simulink model "sistema_completo_discretizado"  (R2023b)
settings: Solver=VariableStepAuto  StartTime=0.0  StopTime=10.0  RelTol=1e-3
values from neighbouring files (symbols this model uses):
  alpha_Cu = 3.9e-3    (= 0.0039)    [controlador_foc_simulink.m]    (also in parametros_planta.m; params_subsistema_termico.m; sistema_completo_en_codigo.m)
  ba_num = Jeq_ctrl*n_pid*wn_pid    (= 0.0395694444444)    [controlador_foc_simulink.m]    (also in sistema_completo_en_codigo.m)
  beq_nom = bm + bl_nom/r^2    (= 2.19444444444e-05)    [parametros_planta.m]    (also in params_subsistema_mecanico.m; sistema_completo_en_codigo.m)
  Cts = 0.818    [parametros_planta.m]    (also in params_subsistema_termico.m)
  g = 9.80665    [controlador_foc_simulink.m]    (also in parametros_planta.m; params_subsistema_mecanico.m; sistema_completo_en_codigo.m)
  Jeq_nom = Jm + Jl_nom/r^2    (= 1.97847222222e-05)    [params_subsistema_mecanico.m]    (also in sistema_completo_en_codigo.m)
  kg_eq_nom = g*kl_nom/r    (= 0.0204305208333)    [params_subsistema_mecanico.m]    (also in sistema_completo_en_codigo.m)
  kl_nom = m*Lcm + ml_nom*Ll    (= 0.25)    [controlador_foc_simulink.m]    (also in params_subsistema_mecanico.m; sistema_completo_en_codigo.m)
  Ksa_num = Jeq_ctrl*n_pid*wn_pid^2    (= 31.6555555556)    [controlador_foc_simulink.m]    (also in sistema_completo_en_codigo.m)
  Ksia_num = Jeq_ctrl*wn_pid^3    (= 10129.7777778)    [controlador_foc_simulink.m]    (also in sistema_completo_en_codigo.m)
  L_d = 6.6e-3    (= 0.0066)    [controlador_foc_simulink.m]    (also in params_subsistema_electromagnetico.m; sistema_completo_en_codigo.m)
  L_l = 0.8e-3    (= 0.0008)    [controlador_foc_simulink.m]    (also in params_subsistema_electromagnetico.m; sistema_completo_en_codigo.m)
  L_q = 5.8e-3    (= 0.0058)    [controlador_foc_simulink.m]    (also in params_subsistema_electromagnetico.m; sistema_completo_en_codigo.m)
  lambda_m = 0.016    [controlador_foc_simulink.m]    (also in parametros_planta.m; params_subsistema_electromagnetico.m; sistema_completo_en_codigo.m)
  Pp = 3    [controlador_foc_simulink.m]    (also in parametros_planta.m; params_subsistema_electromagnetico.m; sistema_completo_en_codigo.m)
  r = 120.0    (= 120)    [controlador_foc_simulink.m]    (also in parametros_planta.m; params_subsistema_mecanico.m; sistema_completo_en_codigo.m)
  Rs_REF = 1.02    [controlador_foc_simulink.m]    (also in parametros_planta.m; params_subsistema_termico.m; sistema_completo_en_codigo.m)
  Rts_amb = 146.7    [parametros_planta.m]    (also in params_subsistema_termico.m)
  Tamb = Tamb_max    (= 40)    [parametros_planta.m]    (also in params_subsistema_termico.m; sistema_completo_en_codigo.m)
  Ts = interp_ts(Ts_ts,t)    [calcular_metricas_operacion.m]
  Ts_REF = 20.0    (= 20)    [controlador_foc_simulink.m]    (also in parametros_planta.m; params_subsistema_termico.m; sistema_completo_en_codigo.m)
undefined symbols (not defined in the file or in its folder): A_iabc, A_pos, A_T, A_v, B_iabc, B_pos, B_T, B_v, C_iabc, C_pos, C_T, C_v, D_iabc, D_pos, D_T, D_v, DiscIntNeverNeededParam, K_ei_ext_agresivo, K_eth_ext_agresivo, K_ew_ext_agresivo
settings Model: Creator=Pc  LastModifiedBy=Pc

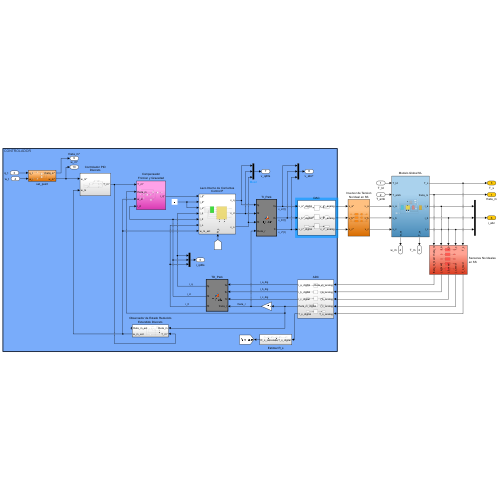
[thumbnail: Simulink's stored preview of the top-level diagram]
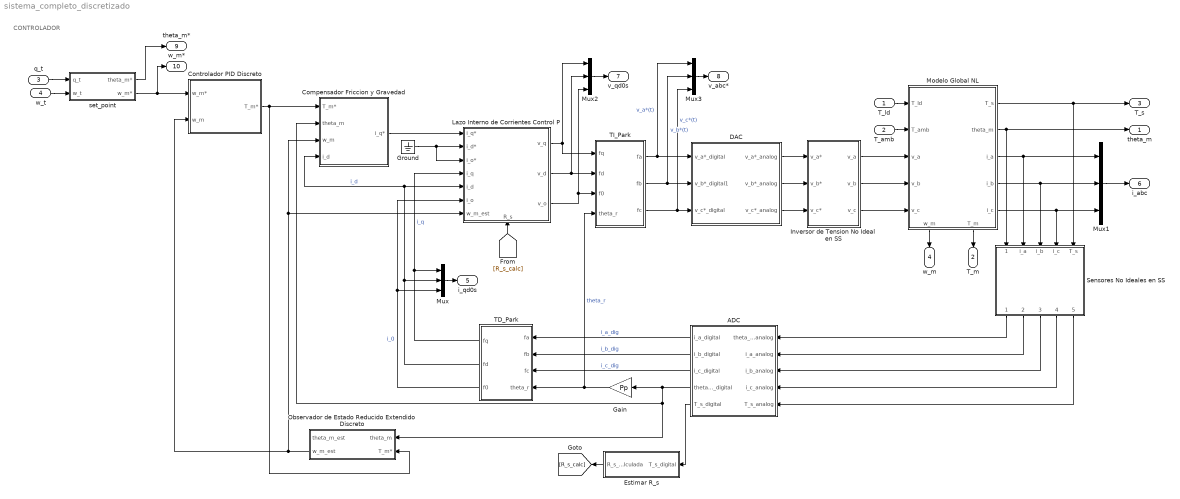
== system sistema_completo_discretizado ==
  note: CONTROLADOR
  T_ld : Inport
  T_amb : Inport  Port=2
  q_t : Inport  Port=3
  w_t : Inport  Port=4
  " ADC" : Subsystem
  Compensador Friccion y Gravedad : Subsystem
  Controlador PID Discreto : Subsystem
  DAC : Subsystem
  Estimar R_s : Subsystem
  Gain : Gain  Gain=Pp
  Ground : Ground
  Inversor de Tension No Ideal en SS : Subsystem
  Lazo Interno de Corrientes Control P : Subsystem
      settings: PortSchema="{\"entries\":[{\"content\":{\"sides\":[{\"content\":{\"connectorIds\":[\"In1\",\"In2\",\"In3\",\"In4\",\"In5\",\"In6\",\"In7\"]},\"type\":\"ConnectorPlacement.EquallySpacedRectSide\",\"uuid\":\"003130de-7086-42b2-88ab-1550be464119\"},{\"content\":{\"connectorIds\":[\"Out1\",\"Out2\",\"Out3\"],\"side\":\"RIGHT\"},\"type\":\"ConnectorPlacement.EquallySpacedRectSide\",\"uuid\":\"1ef26d10-ae91-4351-8dbc-50b579db1e66\"},{\"content\":{\"side\":\"TOP\"},\"type\":\"ConnectorPlacement.EquallySpacedRectSide\",\"uuid\":\"f8d5b360-b304-4c62-a3c0-e85b3671d199\"},{\"content\":{\"connectorIds\":[\"In8\"],\"side\":\"BOTTOM\"},\"type\":\"ConnectorPlacement.EquallySpacedRectSide\",\"uuid\":\"ca7bddea-434a-49b1-aeae-36f1f1b68346\"}]},\"type\":\"ConnectorPlacement.EquallySpacedConnector\",\"uuid\":\"97d0594b-d096-4b47-8675-ea576c5ffe32\"}],\"packageUris\":[\"http://schema.mathworks.com/mf0/Connector/R2020b\"],\"version\":\"1.0\"}"
  Modelo Global NL : Subsystem
      settings: PortSchema="{\"entries\":[{\"content\":{\"sides\":[{\"content\":{\"connectorIds\":[\"In1\",\"In2\",\"In3\",\"In4\",\"In5\"]},\"type\":\"ConnectorPlacement.EquallySpacedRectSide\",\"uuid\":\"386252be-5f39-4928-a151-52e681895a84\"},{\"content\":{\"connectorIds\":[\"Out1\",\"Out2\",\"Out3\",\"Out4\",\"Out5\"],\"side\":\"RIGHT\"},\"type\":\"ConnectorPlacement.EquallySpacedRectSide\",\"uuid\":\"aee83b90-e95b-4477-b157-a5534e7c5e6c\"},{\"content\":{\"side\":\"TOP\"},\"type\":\"ConnectorPlacement.EquallySpacedRectSide\",\"uuid\":\"e739b3f7-cae1-4498-b396-d13f7405e232\"},{\"content\":{\"connectorIds\":[\"Out6\",\"Out7\"],\"side\":\"BOTTOM\"},\"type\":\"ConnectorPlacement.EquallySpacedRectSide\",\"uuid\":\"86304fed-22cd-46a2-87e5-e7bae1c5cedf\"}]},\"type\":\"ConnectorPlacement.EquallySpacedConnector\",\"uuid\":\"c0eb110b-b212-4702-a1d5-9ec3ac2ff196\"}],\"packageUris\":[\"http://schema.mathworks.com/mf0/Connector/R2020b\"],\"version\":\"1.0\"}"
  Mux{,1..3} (4 alike) : Mux  Inputs=3
  Observador de Estado Reducido Extendido Discreto : Subsystem
  Sensores No Ideales en SS : Subsystem
  TD_Park : MATLAB Function  TreatAsAtomicUnit=on
  TI_Park : MATLAB Function  TreatAsAtomicUnit=on
  set_point : Subsystem
  theta_m : Outport
  T_m : Outport  Port=2
  T_s : Outport  Port=3
  w_m : Outport  Port=4
  i_qd0s : Outport  Port=5
  i_abc : Outport  Port=6
  v_qd0s : Outport  Port=7
  v_abc* : Outport  Port=8
  theta_m* : Outport  Port=9
  w_m* : Outport  Port=10
  wires:
  Inversor de Tension No Ideal en SS/3(v_c) -> Modelo Global NL/5(v_c)
  w_t/1 -> set_point/2(w_t)
  Modelo Global NL/6(w_m) -> w_m/1
  q_t/1 -> set_point/1(q_t)
  Mux1/1 -> i_abc/1
  Ground/1 -> Lazo Interno de Corrientes Control P/3(i_o*), Lazo Interno de Corrientes Control P/2(i_d*)
  T_ld/1 -> Modelo Global NL/1(T_ld)
  TI_Park/2(fb) -> DAC/2(v_b*_digital1), Mux3/2  "v_b*(t)"
  TD_Park/3(f0) -> Mux/3, Lazo Interno de Corrientes Control P/6(i_o)  "i_0"
  Modelo Global NL/3(i_a) -> Mux1/1, Sensores No Ideales en SS/2(i_a)
  TI_Park/3(fc) -> DAC/3(v_c*_digital), Mux3/3  "v_c*(t)"
  T_amb/1 -> Modelo Global NL/2(T_amb)
  Modelo Global NL/5(i_c) -> Mux1/3, Sensores No Ideales en SS/4(i_c)
  Mux3/1 -> v_abc*/1
  TD_Park/1(fq) -> Mux/1, Lazo Interno de Corrientes Control P/4(i_q)  "i_q"
  Sensores No Ideales en SS/1(theta_m_med) -> " ADC"/1(theta_m_analog)
  Gain/1 -> TD_Park/4(theta_r), TI_Park/4(theta_r)  "theta_r"
  Modelo Global NL/4(i_b) -> Mux1/2, Sensores No Ideales en SS/3(i_b)
  set_point/1(theta_m*) -> theta_m*/1
  Inversor de Tension No Ideal en SS/1(v_a) -> Modelo Global NL/3(v_a)
  Modelo Global NL/7(T_m) -> T_m/1
  Mux2/1 -> v_qd0s/1
  TI_Park/1(fa) -> DAC/1(v_a*_digital), Mux3/1  "v_a*(t)"
  TD_Park/2(fd) -> Compensador Friccion y Gravedad/4(i_d), Lazo Interno de Corrientes Control P/5(i_d), Mux/2  "i_d"
  Mux/1 -> i_qd0s/1
  Inversor de Tension No Ideal en SS/2(v_b) -> Modelo Global NL/4(v_b)
  Modelo Global NL/1(T_s) -> Sensores No Ideales en SS/5(T_s), T_s/1
  Modelo Global NL/2(theta_m) -> theta_m/1, Sensores No Ideales en SS/1(theta_m)
  Sensores No Ideales en SS/2(i_a_med) -> " ADC"/2(i_a_analog)
  Sensores No Ideales en SS/3(i_b_med) -> " ADC"/3(i_b_analog)
  Sensores No Ideales en SS/4(i_c_med) -> " ADC"/4(i_c_analog)
  DAC/3(v_c*_analog) -> Inversor de Tension No Ideal en SS/3(v_c*)
  DAC/2(v_b*_analog) -> Inversor de Tension No Ideal en SS/2(v_b*)
  DAC/1(v_a*_analog) -> Inversor de Tension No Ideal en SS/1(v_a*)
  " ADC"/1(i_a_digital) -> TD_Park/1(fa)  "i_a_dig"
  " ADC"/2(i_b_digital) -> TD_Park/2(fb)  "i_b_dig"
  " ADC"/3(i_c_digital) -> TD_Park/3(fc)  "i_c_dig"
  Sensores No Ideales en SS/5(T_s_med) -> " ADC"/5(T_s_analog)
  Lazo Interno de Corrientes Control P/1(v_q) -> TI_Park/1(fq), Mux2/1
  Lazo Interno de Corrientes Control P/2(v_d) -> TI_Park/2(fd), Mux2/2
  Lazo Interno de Corrientes Control P/3(v_o) -> TI_Park/3(f0), Mux2/3
  Compensador Friccion y Gravedad/1(i_q*) -> Lazo Interno de Corrientes Control P/1(i_q*)
  " ADC"/5(T_s_digital) -> Estimar R_s/1(T_s_digital)
  [R_s_calc] -> Lazo Interno de Corrientes Control P/8(R_s)
  Estimar R_s/1(R_s_calculada) -> [R_s_calc]
  Controlador PID Discreto/1(T_m*) -> Observador de Estado Reducido Extendido Discreto/2(T_m*), Compensador Friccion y Gravedad/1(T_m*)
  set_point/2(w_m*) -> Controlador PID Discreto/1(w_m*), w_m*/1
  Observador de Estado Reducido Extendido Discreto/2(w_m_est) -> Controlador PID Discreto/2(w_m), Lazo Interno de Corrientes Control P/7(w_m_est), Compensador Friccion y Gravedad/3(w_m)
  " ADC"/4(theta_m_digital) -> Gain/1, Observador de Estado Reducido Extendido Discreto/1(theta_m), Compensador Friccion y Gravedad/2(theta_m)

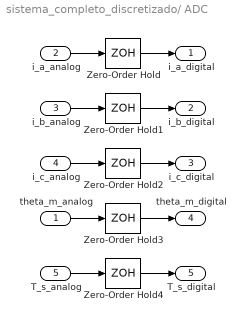
== system sistema_completo_discretizado/ ADC ==
  theta_m_analog : Inport
  i_a_analog : Inport  Port=2
  i_b_analog : Inport  Port=3
  i_c_analog : Inport  Port=4
  T_s_analog : Inport  Port=5
  Zero-Order Hold{,1..4} (5 alike) : ZeroOrderHold  SampleTime=Ts
  i_a_digital : Outport
  i_b_digital : Outport  Port=2
  i_c_digital : Outport  Port=3
  theta_m_digital : Outport  Port=4
  T_s_digital : Outport  Port=5
  wires:
  theta_m_analog/1 -> Zero-Order Hold3/1
  i_a_analog/1 -> Zero-Order Hold/1
  Zero-Order Hold/1 -> i_a_digital/1
  i_c_analog/1 -> Zero-Order Hold2/1
  i_b_analog/1 -> Zero-Order Hold1/1
  T_s_analog/1 -> Zero-Order Hold4/1
  Zero-Order Hold1/1 -> i_b_digital/1
  Zero-Order Hold2/1 -> i_c_digital/1
  Zero-Order Hold3/1 -> theta_m_digital/1
  Zero-Order Hold4/1 -> T_s_digital/1

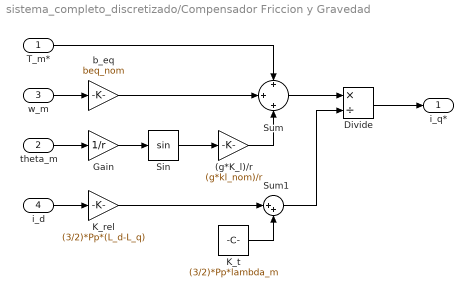
== system sistema_completo_discretizado/Compensador Friccion y Gravedad ==
  T_m* : Inport
  theta_m : Inport  Port=2
  w_m : Inport  Port=3
  i_d : Inport  Port=4
  (g*K_l)/r : Gain  Gain=(g*kl_nom)/r
  Divide : Product  Inputs=*/
  Gain : Gain  Gain=1/r
  K_rel : Gain  Gain=(3/2)*Pp*(L_d-L_q)
  K_t : Constant  Value=(3/2)*Pp*lambda_m
  Sin : Trigonometry
  Sum : Sum  Inputs=+|+|+
  Sum1 : Sum  Inputs=|++
  b_eq : Gain  Gain=beq_nom
  i_q* : Outport
  wires:
  i_d/1 -> K_rel/1
  T_m*/1 -> Sum/1
  Sin/1 -> (g*K_l)/r/1
  K_t/1 -> Sum1/2
  (g*K_l)/r/1 -> Sum/3
  Sum1/1 -> Divide/2
  Gain/1 -> Sin/1
  b_eq/1 -> Sum/2
  K_rel/1 -> Sum1/1
  w_m/1 -> b_eq/1
  Sum/1 -> Divide/1
  Divide/1 -> i_q*/1
  theta_m/1 -> Gain/1

== system sistema_completo_discretizado/Controlador PID Discreto ==
  w_m* : Inport
  w_m : Inport  Port=2
  Discrete-Time Integrator : DiscreteIntegrator  IntegratorMethod=Integration: Trapezoidal  SampleTime=-1  ICPrevOutput=DiscIntNeverNeededParam  ICPrevScaledInput=DiscIntNeverNeededParam
  Discrete-Time Integrator1 : DiscreteIntegrator  IntegratorMethod=Integration: Trapezoidal  SampleTime=-1  ICPrevOutput=DiscIntNeverNeededParam  ICPrevScaledInput=DiscIntNeverNeededParam
  Ksa : Gain  Gain=Ksa_num
  Ksia : Gain  Gain=Ksia_num
  Sum : Sum  Inputs=++|
  Sum1 : Sum  Inputs=+|+|+
  ba : Gain  Gain=ba_num
  T_m* : Outport
  wires:
  Sum1/1 -> T_m*/1
  ba/1 -> Sum1/3  "D"
  Sum/1 -> ba/1, Discrete-Time Integrator/1  "err_w_m"
  Discrete-Time Integrator1/1 -> Ksia/1
  w_m*/1 -> Sum/1
  Discrete-Time Integrator/1 -> Ksa/1, Discrete-Time Integrator1/1
  w_m/1 -> Sum/2
  Ksia/1 -> Sum1/1  "I"
  Ksa/1 -> Sum1/2  "P"

== system sistema_completo_discretizado/DAC ==
  v_a*_digital : Inport
  v_b*_digital1 : Inport  Port=2
  v_c*_digital : Inport  Port=3
  First Order Hold1 : FirstOrderHold  ErrorTolerance=inf  AllowContinuousInput=on
  First Order Hold2 : FirstOrderHold  ErrorTolerance=inf  AllowContinuousInput=on
  First Order Hold4 : FirstOrderHold  ErrorTolerance=inf  AllowContinuousInput=on
  v_a*_analog : Outport
  v_b*_analog : Outport  Port=2
  v_c*_analog : Outport  Port=3
  wires:
  v_c*_digital/1 -> First Order Hold2/1
  v_b*_digital1/1 -> First Order Hold1/1
  v_a*_digital/1 -> First Order Hold4/1
  First Order Hold4/1 -> v_a*_analog/1
  First Order Hold1/1 -> v_b*_analog/1
  First Order Hold2/1 -> v_c*_analog/1

== system sistema_completo_discretizado/Estimar R_s ==
  T_s_digital : Inport
  Constant3 : Constant
  Rs_ref : Gain  Gain=Rs_REF
  Sum3 : Sum  Inputs=|+-
  Sum4 : Sum  Inputs=|++
  Ts_ref : Constant  Value=Ts_REF
  alpha_Cu : Gain  Gain=alpha_Cu
  R_s_calculada : Outport
  wires:
  Ts_ref/1 -> Sum3/2
  T_s_digital/1 -> Sum3/1
  Constant3/1 -> Sum4/2
  Rs_ref/1 -> R_s_calculada/1  "R_s"
  Sum4/1 -> Rs_ref/1
  Sum3/1 -> alpha_Cu/1
  alpha_Cu/1 -> Sum4/1

== system sistema_completo_discretizado/Inversor de Tension No Ideal en SS ==
  v_a* : Inport
  v_b* : Inport  Port=2
  v_c* : Inport  Port=3
  Saturation : Saturate  UpperLimit=39.19  LowerLimit=-39.19
  Saturation1 : Saturate  UpperLimit=39.19  LowerLimit=-39.19
  Saturation2 : Saturate  UpperLimit=39.19  LowerLimit=-39.19
  State-Space : StateSpace  A=A_v  B=B_v  C=C_v  D=D_v  InitialCondition=0
  State-Space1 : StateSpace  A=A_v  B=B_v  C=C_v  D=D_v  InitialCondition=0
  State-Space2 : StateSpace  A=A_v  B=B_v  C=C_v  D=D_v  InitialCondition=0
  v_a : Outport
  v_b : Outport  Port=2
  v_c : Outport  Port=3
  wires:
  Saturation1/1 -> v_b/1
  State-Space1/1 -> Saturation1/1
  Saturation/1 -> v_a/1
  v_c*/1 -> State-Space2/1
  Saturation2/1 -> v_c/1
  State-Space2/1 -> Saturation2/1
  v_b*/1 -> State-Space1/1
  State-Space/1 -> Saturation/1
  v_a*/1 -> State-Space/1

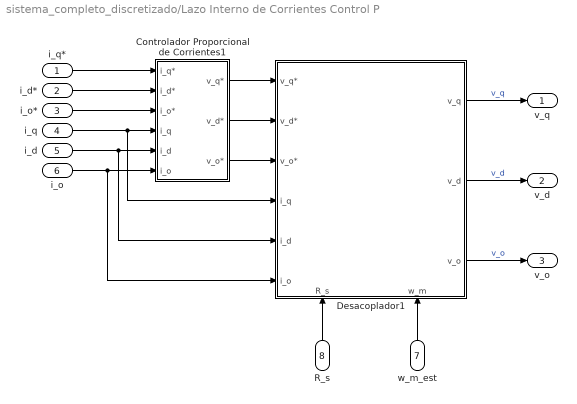
== system sistema_completo_discretizado/Lazo Interno de Corrientes Control P ==
  i_q* : Inport
  i_d* : Inport  Port=2
  i_o* : Inport  Port=3
  i_q : Inport  Port=4
  i_d : Inport  Port=5
  i_o : Inport  Port=6
  w_m_est : Inport  Port=7
  R_s : Inport  Port=8
  Controlador Proporcional de Corrientes1 : Subsystem
  Desacoplador1 : Subsystem
      settings: PortSchema="{\"entries\":[{\"content\":{\"sides\":[{\"content\":{\"connectorIds\":[\"In1\",\"In2\",\"In3\",\"In4\",\"In5\",\"In6\"]},\"type\":\"ConnectorPlacement.EquallySpacedRectSide\",\"uuid\":\"003130de-7086-42b2-88ab-1550be464119\"},{\"content\":{\"connectorIds\":[\"Out1\",\"Out2\",\"Out3\"],\"side\":\"RIGHT\"},\"type\":\"ConnectorPlacement.EquallySpacedRectSide\",\"uuid\":\"1ef26d10-ae91-4351-8dbc-50b579db1e66\"},{\"content\":{\"side\":\"TOP\"},\"type\":\"ConnectorPlacement.EquallySpacedRectSide\",\"uuid\":\"f8d5b360-b304-4c62-a3c0-e85b3671d199\"},{\"content\":{\"connectorIds\":[\"In7\",\"In8\"],\"side\":\"BOTTOM\"},\"type\":\"ConnectorPlacement.EquallySpacedRectSide\",\"uuid\":\"ed3aa2b2-0c88-4f8f-b202-0aa60a8551ab\"}]},\"type\":\"ConnectorPlacement.EquallySpacedConnector\",\"uuid\":\"97d0594b-d096-4b47-8675-ea576c5ffe32\"}],\"packageUris\":[\"http://schema.mathworks.com/mf0/Connector/R2020b\"],\"version\":\"1.0\"}"
  v_q : Outport
  v_d : Outport  Port=2
  v_o : Outport  Port=3
  wires:
  Desacoplador1/3(v_o) -> v_o/1  "v_o"
  Controlador Proporcional de Corrientes1/1(v_q*) -> Desacoplador1/1(v_q*)
  Desacoplador1/1(v_q) -> v_q/1  "v_q"
  w_m_est/1 -> Desacoplador1/8(w_m)
  Controlador Proporcional de Corrientes1/3(v_o*) -> Desacoplador1/3(v_o*)
  i_d/1 -> Controlador Proporcional de Corrientes1/5(i_d), Desacoplador1/5(i_d)
  i_q/1 -> Controlador Proporcional de Corrientes1/4(i_q), Desacoplador1/4(i_q)
  i_o/1 -> Controlador Proporcional de Corrientes1/6(i_o), Desacoplador1/6(i_o)
  i_d*/1 -> Controlador Proporcional de Corrientes1/2(i_d*)
  i_q*/1 -> Controlador Proporcional de Corrientes1/1(i_q*)
  i_o*/1 -> Controlador Proporcional de Corrientes1/3(i_o*)
  Controlador Proporcional de Corrientes1/2(v_d*) -> Desacoplador1/2(v_d*)
  R_s/1 -> Desacoplador1/7(R_s)
  Desacoplador1/2(v_d) -> v_d/1  "v_d"

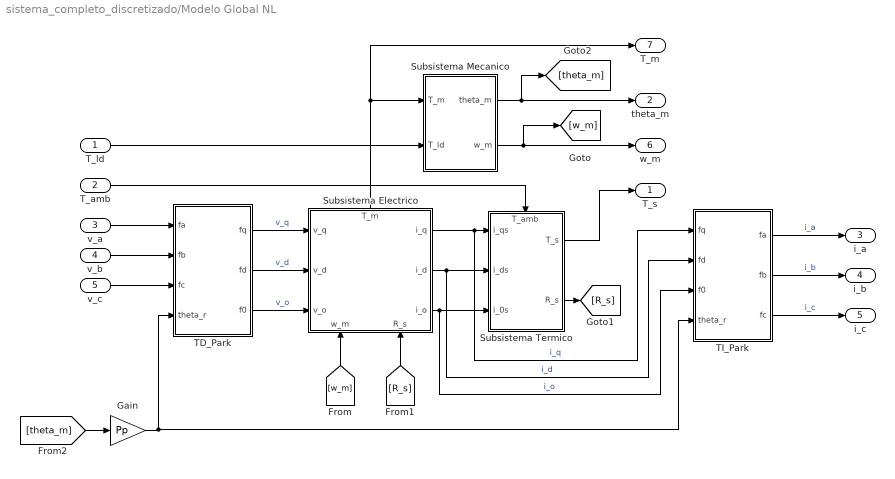
== system sistema_completo_discretizado/Modelo Global NL ==
  T_ld : Inport
  T_amb : Inport  Port=2
  v_a : Inport  Port=3
  v_b : Inport  Port=4
  v_c : Inport  Port=5
  Gain : Gain  Gain=Pp
  Subsistema Electrico : Subsystem
      settings: PortSchema="{\"entries\":[{\"content\":{\"sides\":[{\"content\":{\"connectorIds\":[\"In1\",\"In2\",\"In3\"]},\"type\":\"ConnectorPlacement.EquallySpacedRectSide\",\"uuid\":\"c7eb63ae-4015-4be9-a2f8-5ddbad38e871\"},{\"content\":{\"connectorIds\":[\"Out1\",\"Out2\",\"Out3\"],\"side\":\"RIGHT\"},\"type\":\"ConnectorPlacement.EquallySpacedRectSide\",\"uuid\":\"ed205027-9864-417a-9d2b-6eeb723ffec2\"},{\"content\":{\"connectorIds\":[\"Out4\"],\"side\":\"TOP\"},\"type\":\"ConnectorPlacement.EquallySpacedRectSide\",\"uuid\":\"5c5dee03-5728-4212-8fc2-a453d3484329\"},{\"content\":{\"connectorIds\":[\"In4\",\"In5\"],\"side\":\"BOTTOM\"},\"type\":\"ConnectorPlacement.EquallySpacedRectSide\",\"uuid\":\"494df340-b6d5-4f09-932e-9dbff39af1cf\"}]},\"type\":\"ConnectorPlacement.EquallySpacedConnector\",\"uuid\":\"0eeaea4c-3d80-4ebb-8c27-59b1b18764e9\"}],\"packageUris\":[\"http://schema.mathworks.com/mf0/Connector/R2020b\"],\"version\":\"1.0\"}"
  Subsistema Mecanico : Subsystem
  Subsistema Termico : Subsystem
      settings: PortSchema="{\"entries\":[{\"content\":{\"sides\":[{\"content\":{\"connectorIds\":[\"In1\",\"In2\",\"In3\"]},\"type\":\"ConnectorPlacement.EquallySpacedRectSide\",\"uuid\":\"5b1848a7-84bd-4673-a3fa-3976b4d0d5b9\"},{\"content\":{\"connectorIds\":[\"Out1\",\"Out2\"],\"side\":\"RIGHT\"},\"type\":\"ConnectorPlacement.EquallySpacedRectSide\",\"uuid\":\"feff3f8a-cd7c-43b1-91c3-7ab01b0b33a6\"},{\"content\":{\"connectorIds\":[\"In4\"],\"side\":\"TOP\"},\"type\":\"ConnectorPlacement.EquallySpacedRectSide\",\"uuid\":\"8de0b1b6-142f-442a-a92f-2baa615c6322\"}]},\"type\":\"ConnectorPlacement.EquallySpacedConnector\",\"uuid\":\"046fcb24-e0d9-4784-a784-7e36f9acbfbc\"}],\"packageUris\":[\"http://schema.mathworks.com/mf0/Connector/R2020b\"],\"version\":\"1.0\"}"
  TD_Park : MATLAB Function  TreatAsAtomicUnit=on
  TI_Park : MATLAB Function  TreatAsAtomicUnit=on
  T_s : Outport
  theta_m : Outport  Port=2
  i_a : Outport  Port=3
  i_b : Outport  Port=4
  i_c : Outport  Port=5
  w_m : Outport  Port=6
  T_m : Outport  Port=7
  wires:
  Subsistema Mecanico/1(theta_m) -> theta_m/1, [theta_m]
  TD_Park/2(fd) -> Subsistema Electrico/2(v_d)  "v_d"
  Subsistema Termico/1(T_s) -> T_s/1
  TD_Park/3(f0) -> Subsistema Electrico/3(v_o)  "v_o"
  Subsistema Mecanico/2(w_m) -> w_m/1, [w_m]
  [R_s] -> Subsistema Electrico/5(R_s)
  TI_Park/1(fa) -> i_a/1  "i_a"
  TD_Park/1(fq) -> Subsistema Electrico/1(v_q)  "v_q"
  Subsistema Electrico/4(T_m) -> T_m/1, Subsistema Mecanico/1(T_m)
  v_c/1 -> TD_Park/3(fc)
  Subsistema Electrico/2(i_d) -> Subsistema Termico/2(i_ds), TI_Park/2(fd)  "i_d"
  Subsistema Termico/2(R_s) -> [R_s]
  T_amb/1 -> Subsistema Termico/4(T_amb)
  T_ld/1 -> Subsistema Mecanico/2(T_ld)
  Subsistema Electrico/3(i_o) -> Subsistema Termico/3(i_0s), TI_Park/3(f0)  "i_o"
  TI_Park/2(fb) -> i_b/1  "i_b"
  Subsistema Electrico/1(i_q) -> TI_Park/1(fq), Subsistema Termico/1(i_qs)  "i_q"
  v_a/1 -> TD_Park/1(fa)
  v_b/1 -> TD_Park/2(fb)
  [w_m] -> Subsistema Electrico/4(w_m)
  TI_Park/3(fc) -> i_c/1  "i_c"
  [theta_m] -> Gain/1
  Gain/1 -> TD_Park/4(theta_r), TI_Park/4(theta_r)

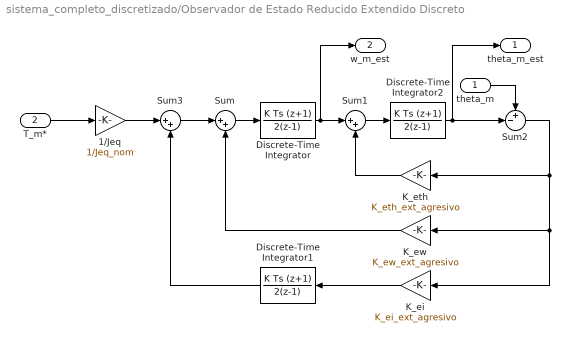
== system sistema_completo_discretizado/Observador de Estado Reducido Extendido Discreto ==
  theta_m : Inport
  T_m* : Inport  Port=2
  1/Jeq : Gain  Gain=1/Jeq_nom
  Discrete-Time Integrator : DiscreteIntegrator  IntegratorMethod=Integration: Trapezoidal  SampleTime=-1  ICPrevOutput=DiscIntNeverNeededParam  ICPrevScaledInput=DiscIntNeverNeededParam
  Discrete-Time Integrator1 : DiscreteIntegrator  IntegratorMethod=Integration: Trapezoidal  SampleTime=-1  ICPrevOutput=DiscIntNeverNeededParam  ICPrevScaledInput=DiscIntNeverNeededParam
  Discrete-Time Integrator2 : DiscreteIntegrator  IntegratorMethod=Integration: Trapezoidal  SampleTime=-1  ICPrevOutput=DiscIntNeverNeededParam  ICPrevScaledInput=DiscIntNeverNeededParam
  K_ei : Gain  Gain=K_ei_ext_agresivo
  K_eth : Gain  Gain=K_eth_ext_agresivo
  K_ew : Gain  Gain=K_ew_ext_agresivo
  Sum : Sum  Inputs=|++
  Sum1 : Sum  Inputs=|++
  Sum2 : Sum  Inputs=+-|
  Sum3 : Sum  Inputs=|++
  theta_m_est : Outport
  w_m_est : Outport  Port=2
  wires:
  K_eth/1 -> Sum1/2
  Discrete-Time Integrator2/1 -> Sum2/2, theta_m_est/1
  Sum3/1 -> Sum/1
  Discrete-Time Integrator/1 -> w_m_est/1, Sum1/1
  K_ew/1 -> Sum/2
  Sum2/1 -> K_ei/1, K_ew/1, K_eth/1
  1/Jeq/1 -> Sum3/1
  Sum/1 -> Discrete-Time Integrator/1
  theta_m/1 -> Sum2/1
  T_m*/1 -> 1/Jeq/1
  Discrete-Time Integrator1/1 -> Sum3/2
  Sum1/1 -> Discrete-Time Integrator2/1
  K_ei/1 -> Discrete-Time Integrator1/1

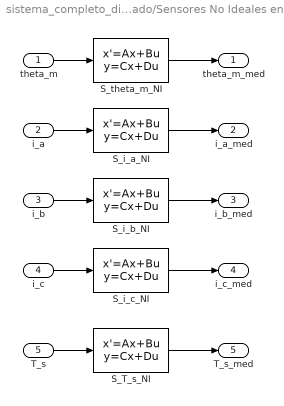
== system sistema_completo_discretizado/Sensores No Ideales en SS ==
  theta_m : Inport
  i_a : Inport  Port=2
  i_b : Inport  Port=3
  i_c : Inport  Port=4
  T_s : Inport  Port=5
  S_T_s_NI : StateSpace  A=A_T  B=B_T  C=C_T  D=D_T  InitialCondition=0
  S_i_a_NI : StateSpace  A=A_iabc  B=B_iabc  C=C_iabc  D=D_iabc  InitialCondition=0
  S_i_b_NI : StateSpace  A=A_iabc  B=B_iabc  C=C_iabc  D=D_iabc  InitialCondition=0
  S_i_c_NI : StateSpace  A=A_iabc  B=B_iabc  C=C_iabc  D=D_iabc  InitialCondition=0
  S_theta_m_NI : StateSpace  A=A_pos  B=B_pos  C=C_pos  D=D_pos  InitialCondition=0
  theta_m_med : Outport
  i_a_med : Outport  Port=2
  i_b_med : Outport  Port=3
  i_c_med : Outport  Port=4
  T_s_med : Outport  Port=5
  wires:
  S_i_b_NI/1 -> i_b_med/1
  i_b/1 -> S_i_b_NI/1
  T_s/1 -> S_T_s_NI/1
  i_c/1 -> S_i_c_NI/1
  S_i_c_NI/1 -> i_c_med/1
  S_T_s_NI/1 -> T_s_med/1
  i_a/1 -> S_i_a_NI/1
  S_theta_m_NI/1 -> theta_m_med/1
  theta_m/1 -> S_theta_m_NI/1
  S_i_a_NI/1 -> i_a_med/1

== system sistema_completo_discretizado/set_point ==
  q_t : Inport
  w_t : Inport  Port=2
  Derivative : Derivative
  Gain : Gain  Gain=r
  Gain1 : Gain  Gain=r
  Integrator : Integrator
  Sum : Sum  Inputs=|++
  Sum1 : Sum  Inputs=|++
  theta_m* : Outport
  w_m* : Outport  Port=2
  wires:
  Gain1/1 -> Derivative/1, Sum/1
  Derivative/1 -> Sum1/1
  Gain/1 -> Integrator/1, Sum1/2
  Integrator/1 -> Sum/2
  Sum/1 -> theta_m*/1
  Sum1/1 -> w_m*/1
  w_t/1 -> Gain/1
  q_t/1 -> Gain1/1

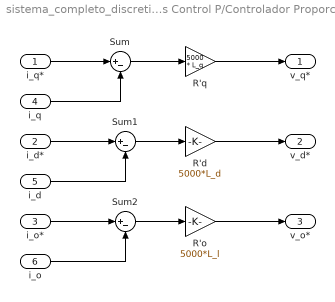
== system sistema_completo_discretizado/Lazo Interno de Corrientes Control P/Controlador Proporcional de Corrientes1 ==
  i_q* : Inport
  i_d* : Inport  Port=2
  i_o* : Inport  Port=3
  i_q : Inport  Port=4
  i_d : Inport  Port=5
  i_o : Inport  Port=6
  R'd : Gain  Gain=5000*L_d
  R'o : Gain  Gain=5000*L_l
  R'q : Gain  Gain=5000 * L_q
  Sum : Sum  Inputs=|+-
  Sum1 : Sum  Inputs=|+-
  Sum2 : Sum  Inputs=|+-
  v_q* : Outport
  v_d* : Outport  Port=2
  v_o* : Outport  Port=3
  wires:
  R'd/1 -> v_d*/1
  i_q/1 -> Sum/2
  i_d*/1 -> Sum1/1
  R'o/1 -> v_o*/1
  i_o*/1 -> Sum2/1
  Sum/1 -> R'q/1
  Sum1/1 -> R'd/1
  i_o/1 -> Sum2/2
  Sum2/1 -> R'o/1
  R'q/1 -> v_q*/1
  i_d/1 -> Sum1/2
  i_q*/1 -> Sum/1

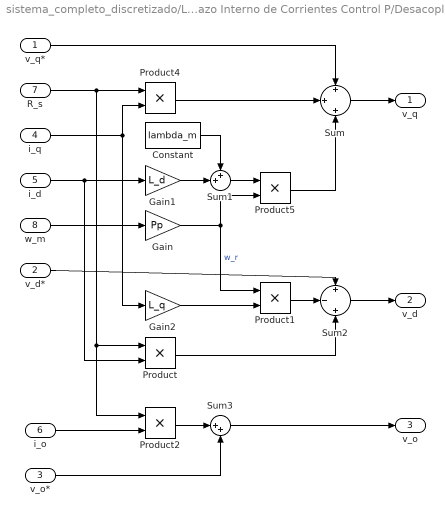
== system sistema_completo_discretizado/Lazo Interno de Corrientes Control P/Desacoplador1 ==
  v_q* : Inport
  v_d* : Inport  Port=2
  v_o* : Inport  Port=3
  i_q : Inport  Port=4
  i_d : Inport  Port=5
  i_o : Inport  Port=6
  R_s : Inport  Port=7
  w_m : Inport  Port=8
  Constant : Constant  Value=lambda_m
  Gain : Gain  Gain=Pp
  Gain1 : Gain  Gain=L_d
  Gain2 : Gain  Gain=L_q
  Product{,1..2,4..5} (5 alike) : Product
  Sum : Sum  Inputs=+|+|+
  Sum1 : Sum  Inputs=++|
  Sum2 : Sum  Inputs=+|-|+
  Sum3 : Sum  Inputs=|++
  v_q : Outport
  v_d : Outport  Port=2
  v_o : Outport  Port=3
  wires:
  R_s/1 -> Product/1, Product2/1, Product4/1
  Product2/1 -> Sum3/1
  v_d*/1 -> Sum2/1
  Gain/1 -> Product1/1, Product5/2  "w_r"
  Gain1/1 -> Sum1/2
  Product/1 -> Sum2/3
  Sum3/1 -> v_o/1
  i_d/1 -> Gain1/1, Product/2
  Product5/1 -> Sum/3
  Product1/1 -> Sum2/2
  Product4/1 -> Sum/2
  v_q*/1 -> Sum/1
  i_q/1 -> Gain2/1, Product4/2
  Sum/1 -> v_q/1
  i_o/1 -> Product2/2
  Sum1/1 -> Product5/1
  Sum2/1 -> v_d/1
  v_o*/1 -> Sum3/2
  w_m/1 -> Gain/1
  Constant/1 -> Sum1/1
  Gain2/1 -> Product1/2

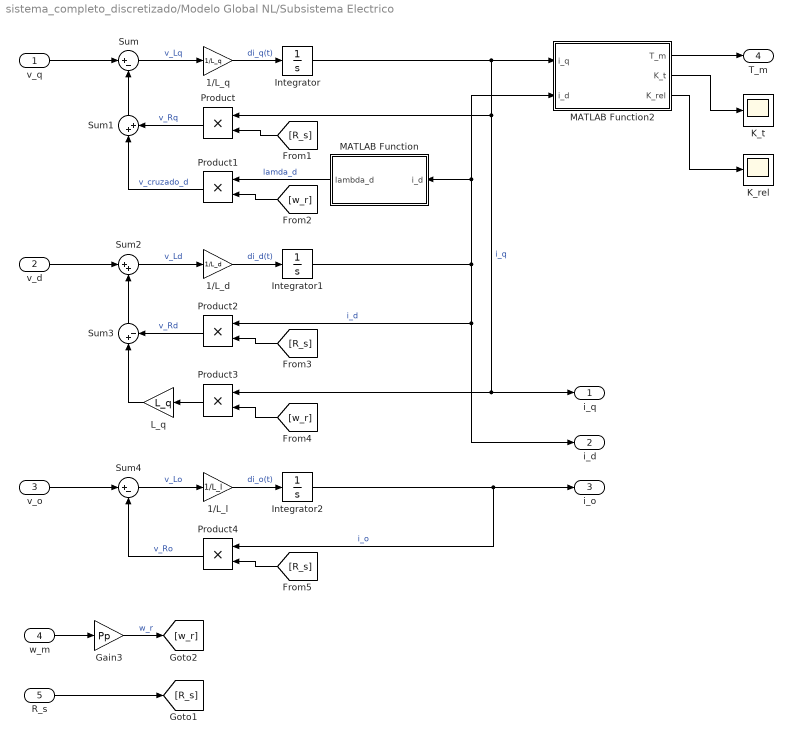
== system sistema_completo_discretizado/Modelo Global NL/Subsistema Electrico ==
  v_q : Inport
  v_d : Inport  Port=2
  v_o : Inport  Port=3
  w_m : Inport  Port=4
  R_s : Inport  Port=5
  1/L_d : Gain  Gain=1/L_d
  1/L_l : Gain  Gain=1/L_l
  1/L_q : Gain  Gain=1/L_q
  Gain3 : Gain  Gain=Pp
  Integrator : Integrator
  Integrator1 : Integrator
  Integrator2 : Integrator
  K_rel : Scope
  K_t : Scope
  L_q : Gain  Gain=L_q
  MATLAB Function : MATLAB Function  TreatAsAtomicUnit=on
  MATLAB Function2 : MATLAB Function  TreatAsAtomicUnit=on
  Product{,1..4} (5 alike) : Product
  Sum : Sum  Inputs=|+-
  Sum1 : Sum  Inputs=|++
  Sum2 : Sum  Inputs=|++
  Sum3 : Sum  Inputs=|+-
  Sum4 : Sum  Inputs=|+-
  i_q : Outport
  i_d : Outport  Port=2
  i_o : Outport  Port=3
  T_m : Outport  Port=4
  wires:
  Integrator/1 -> MATLAB Function2/1(i_q), Product/1, i_q/1, Product3/1  "i_q"
  Sum3/1 -> Sum2/2
  Product1/1 -> Sum1/1  "v_cruzado_d"
  Integrator1/1 -> MATLAB Function2/2(i_d), MATLAB Function/1(i_d), i_d/1, Product2/1  "i_d"
  Sum1/1 -> Sum/2
  1/L_d/1 -> Integrator1/1  "di_d(t)"
  MATLAB Function/1(lambda_d) -> Product1/1  "lamda_d"
  Sum4/1 -> 1/L_l/1  "v_Lo"
  [w_r] -> Product3/2
  Sum/1 -> 1/L_q/1  "v_Lq"
  1/L_l/1 -> Integrator2/1  "di_o(t)"
  Integrator2/1 -> i_o/1, Product4/1  "i_o"
  Product2/1 -> Sum3/2  "v_Rd"
  Product/1 -> Sum1/2  "v_Rq"
  [R_s] -> Product4/2
  Product3/1 -> L_q/1
  1/L_q/1 -> Integrator/1  "di_q(t)"
  Sum2/1 -> 1/L_d/1  "v_Ld"
  v_q/1 -> Sum/1
  [R_s] -> Product/2
  Product4/1 -> Sum4/2  "v_Ro"
  [w_r] -> Product1/2
  [R_s] -> Product2/2
  L_q/1 -> Sum3/1
  v_d/1 -> Sum2/1
  v_o/1 -> Sum4/1
  MATLAB Function2/1(T_m) -> T_m/1
  MATLAB Function2/3(K_rel) -> K_rel/1
  MATLAB Function2/2(K_t) -> K_t/1
  w_m/1 -> Gain3/1
  R_s/1 -> [R_s]
  Gain3/1 -> [w_r]  "w_r"

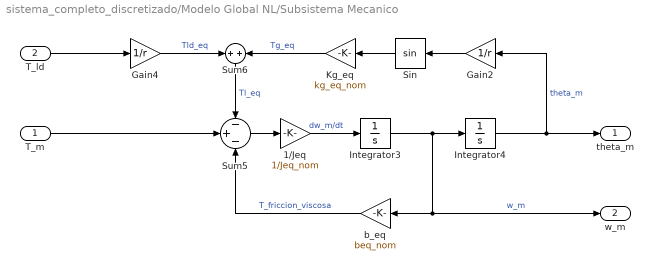
== system sistema_completo_discretizado/Modelo Global NL/Subsistema Mecanico ==
  T_m : Inport
  T_ld : Inport  Port=2
  1/Jeq : Gain  Gain=1/Jeq_nom
  Gain2 : Gain  Gain=1/r
  Gain4 : Gain  Gain=1/r
  Integrator3 : Integrator
  Integrator4 : Integrator
  Kg_eq : Gain  Gain=kg_eq_nom
  Sin : Trigonometry
  Sum5 : Sum  Inputs=-+-
  Sum6 : Sum  Inputs=+|+
  b_eq : Gain  Gain=beq_nom
  theta_m : Outport
  w_m : Outport  Port=2
  wires:
  Sin/1 -> Kg_eq/1
  Gain4/1 -> Sum6/1  "Tld_eq"
  Integrator4/1 -> theta_m/1, Gain2/1  "theta_m"
  Kg_eq/1 -> Sum6/2  "Tg_eq"
  Sum5/1 -> 1/Jeq/1
  b_eq/1 -> Sum5/3  "T_friccion_viscosa"
  T_m/1 -> Sum5/2
  Gain2/1 -> Sin/1
  Sum6/1 -> Sum5/1  "Tl_eq"
  Integrator3/1 -> w_m/1, b_eq/1, Integrator4/1  "w_m"
  T_ld/1 -> Gain4/1
  1/Jeq/1 -> Integrator3/1  "dw_m/dt"

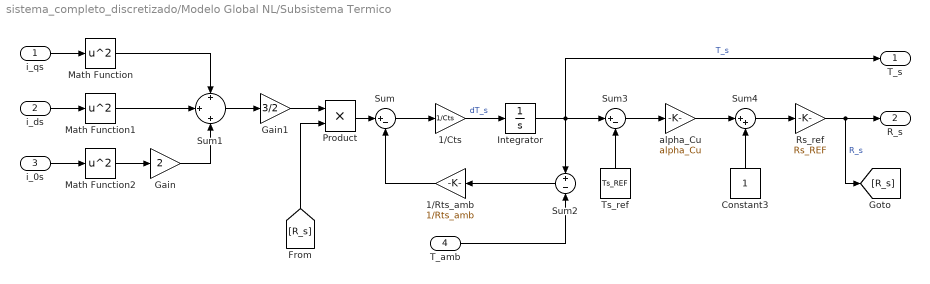
== system sistema_completo_discretizado/Modelo Global NL/Subsistema Termico ==
  i_qs : Inport
  i_ds : Inport  Port=2
  i_0s : Inport  Port=3
  T_amb : Inport  Port=4
  1/Cts : Gain  Gain=1/Cts
  1/Rts_amb : Gain  Gain=1/Rts_amb
  Constant3 : Constant
  Gain : Gain  Gain=2
  Gain1 : Gain  Gain=3/2
  Integrator : Integrator  InitialCondition=Tamb
  Math Function : Math  Operator=square
  Math Function1 : Math  Operator=square
  Math Function2 : Math  Operator=square
  Product : Product
  Rs_ref : Gain  Gain=Rs_REF
  Sum : Sum  Inputs=|+-
  Sum1 : Sum  Inputs=+|+|+
  Sum2 : Sum  Inputs=+-
  Sum3 : Sum  Inputs=|+-
  Sum4 : Sum  Inputs=|++
  Ts_ref : Constant  Value=Ts_REF
  alpha_Cu : Gain  Gain=alpha_Cu
  T_s : Outport
  R_s : Outport  Port=2
  wires:
  1/Cts/1 -> Integrator/1  "dT_s"
  Sum3/1 -> alpha_Cu/1
  Rs_ref/1 -> R_s/1, [R_s]  "R_s"
  Sum4/1 -> Rs_ref/1
  [R_s] -> Product/2
  i_ds/1 -> Math Function1/1
  Constant3/1 -> Sum4/2
  Integrator/1 -> T_s/1, Sum2/1, Sum3/1  "T_s"
  Math Function1/1 -> Sum1/2
  alpha_Cu/1 -> Sum4/1
  Sum2/1 -> 1/Rts_amb/1
  Product/1 -> Sum/1
  i_qs/1 -> Math Function/1
  Sum/1 -> 1/Cts/1
  T_amb/1 -> Sum2/2
  Math Function/1 -> Sum1/1
  i_0s/1 -> Math Function2/1
  1/Rts_amb/1 -> Sum/2
  Ts_ref/1 -> Sum3/2
  Math Function2/1 -> Gain/1
  Gain/1 -> Sum1/3
  Sum1/1 -> Gain1/1
  Gain1/1 -> Product/1

== matlab function sistema_completo_discretizado/Modelo Global NL/TD_Park ==
  data: fa input; fq output; fb input; fc input; theta_r input; fd output; f0 output
function [fq, fd, f0] = T_Park(fa, fb, fc, theta_r)
%#codegen
% Transformada directa de Park: abc -> qd0
% Convención usada:
% fq: eje q
% fd: eje d
% f0: componente homopolar

c1 = cos(theta_r);
c2 = cos(theta_r - 2*pi/3);
c3 = cos(theta_r + 2*pi/3);

s1 = sin(theta_r);
s2 = sin(theta_r - 2*pi/3);
s3 = sin(theta_r + 2*pi/3);

fq = (2/3)*(c1*fa + c2*fb + c3*fc);
fd = (2/3)*(s1*fa + s2*fb + s3*fc);
f0 = (1/3)*(fa + fb + fc);
end

== matlab function sistema_completo_discretizado/Modelo Global NL/Subsistema Electrico/MATLAB Function ==
  data: i_d input; lambda_d output; lambda_m parameter; L_d parameter
function lambda_d = calcular_flujo_d(i_d, lambda_m, L_d)
    % CALCULAR_FLUJO_D Calcula el flujo magnético total concatenado en el eje directo (d).
    %
    % Entradas:
    %   i_d      : Corriente instantánea en el eje d (Señal dinámica de entrada).
    %   lambda_m : Flujo de los imanes permanentes (Parámetro estático).
    %   L_d      : Inductancia del estator en el eje d (Parámetro estático).
    %
    % Salida:
    %   lambda_d : Flujo magnético total en el eje d.

    % Cálculo: Flujo de imanes + Flujo de reacción del inducido
    lambda_d = lambda_m + L_d * i_d;
end

== matlab function sistema_completo_discretizado/Modelo Global NL/Subsistema Electrico/MATLAB Function2 ==
  data: i_q input; i_d input; T_m output; Pp parameter; lambda_m parameter; L_d parameter; L_q parameter; K_t output; K_rel output
function [T_m, K_t, K_rel] = calcular_torque(i_q, i_d, Pp, lambda_m, L_d, L_q)
    % CALCULAR_TORQUE Calcula el torque electromagnético total de la máquina PMSM
    % y sus constantes equivalentes.
    % 
    % Entradas dinámicas (Inports):
    %   i_q      : Corriente en el eje en cuadratura [A].
    %   i_d      : Corriente en el eje directo [A].
    %
    % Parámetros estáticos (Parameters):
    %   P_p      : Número de pares de polos.
    %   lambda_m : Flujo magnético de los imanes permanentes [Wb].
    %   L_d      : Inductancia del eje d [H].
    %   L_q      : Inductancia del eje q [H].
    %
    % Salidas:
    %   T_m      : Torque electromagnético generado [N.m].
    %   K_t      : Constante de torque de alineación [N.m/A].
    %   K_rel    : Constante de torque de reluctancia [N.m/A^2].

    % 1. Cálculo de las constantes 
    K_t = (3/2) * Pp * lambda_m;
    K_rel = (3/2) * Pp * (L_d - L_q);

    % 2. Cálculo del torque electromagnético total
    T_m = K_t * i_q + K_rel * i_d * i_q;
end

== matlab function sistema_completo_discretizado/Modelo Global NL/TI_Park ==
  data: fq input; fa output; fd input; f0 input; theta_r input; fb output; fc output
function [fa, fb, fc] = TI_Park(fq, fd, f0, theta_r)
%#codegen
% Transformada inversa de Park: qd0 -> abc

fa = cos(theta_r)*fq ...
   + sin(theta_r)*fd ...
   + f0;

fb = cos(theta_r - 2*pi/3)*fq ...
   + sin(theta_r - 2*pi/3)*fd ...
   + f0;

fc = cos(theta_r + 2*pi/3)*fq ...
   + sin(theta_r + 2*pi/3)*fd ...
   + f0;
end

== matlab function sistema_completo_discretizado/TD_Park ==
  data: fa input; fq output; fb input; fc input; theta_r input; fd output; f0 output
function [fq, fd, f0] = T_Park(fa, fb, fc, theta_r)
%#codegen
% Transformada directa de Park: abc -> qd0
% Convención usada:
% fq: eje q
% fd: eje d
% f0: componente homopolar

c1 = cos(theta_r);
c2 = cos(theta_r - 2*pi/3);
c3 = cos(theta_r + 2*pi/3);

s1 = sin(theta_r);
s2 = sin(theta_r - 2*pi/3);
s3 = sin(theta_r + 2*pi/3);

fq = (2/3)*(c1*fa + c2*fb + c3*fc);
fd = (2/3)*(s1*fa + s2*fb + s3*fc);
f0 = (1/3)*(fa + fb + fc);
end

== matlab function sistema_completo_discretizado/TI_Park ==
  data: fq input; fa output; fd input; f0 input; theta_r input; fb output; fc output
function [fa, fb, fc] = TI_Park(fq, fd, f0, theta_r)
%#codegen
% Transformada inversa de Park: qd0 -> abc

fa = cos(theta_r)*fq ...
   + sin(theta_r)*fd ...
   + f0;

fb = cos(theta_r - 2*pi/3)*fq ...
   + sin(theta_r - 2*pi/3)*fd ...
   + f0;

fc = cos(theta_r + 2*pi/3)*fq ...
   + sin(theta_r + 2*pi/3)*fd ...
   + f0;
end
